simulink model "Flyback_Converter_Model_2014a"  (R2024a)
settings: Solver=ode3  StartTime=0.0  StopTime=0.25  FixedStep=1e-6  MaxStep=1e-4  RelTol=1e-4
libraries: spsSeriesRLCBranchLib x2, spsCurrentMeasurementLib x2, spsVoltageMeasurementLib x2, spsDiodeLib x1, spsMultimeterLib x1, spsMosfetLib x1, spsLinearTransformerLib x1, spsDCVoltageSourceLib x1, sps_lib x1
settings Model: Creator=A0109971  LastModifiedBy=DELL
settings SolverCC: AlgebraicLoopSolver=TrustRegion
settings DataIOCC: SaveFormat=StructureWithTime  ReturnWorkspaceOutputs=off
settings OptimizationCC: LifeSpan=inf
settings DebuggingCC: UnconnectedInputMsg=warning  UnconnectedOutputMsg=warning  UnconnectedLineMsg=warning  SFExecutionAtInitializationDiag=none  ArithmeticOperatorsInVariantConditions=warning
settings HardwareCC: ProdBitPerSizeT=32  ProdBitPerPtrDiffT=32  ProdWordSize=32  ProdHWDeviceType=Specified
settings SFSimCC: SimUseLocalCustomCode=off  CustomCodeUndefinedFunction=UseInterfaceOnly
settings RTWCC: RTWUseLocalCustomCode=off  GPUComputeCapability=3.5
settings CodeAppCC: StateflowObjectComments=on
settings SimscapeCC: SimscapeNormalizeSystem=off

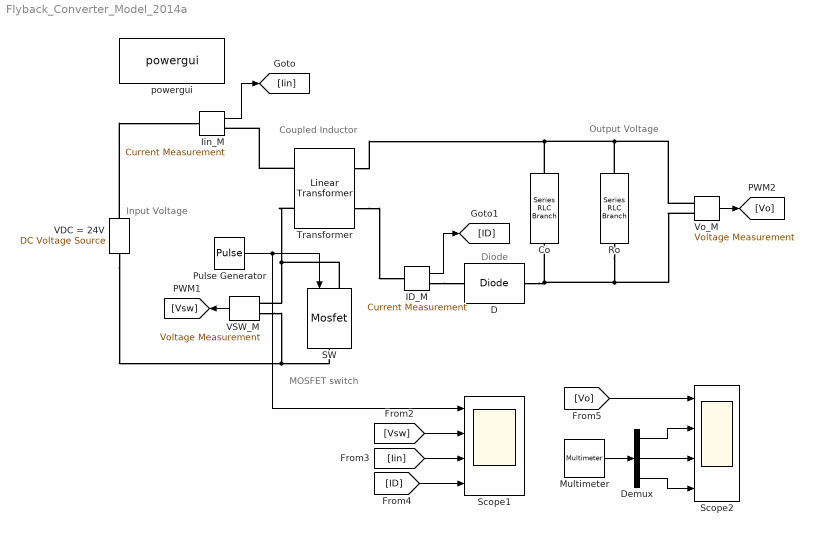
== system Flyback_Converter_Model_2014a ==
  note: Coupled Inductor
  note: Input Voltage
  note: MOSFET switch
  note: Diode
  note: Output Voltage
  Co : spsSeriesRLCBranchLib/Series RLC Branch  LConnTagsString=__new0  RConnTagsString=__new0  BranchType=C  Resistance=1  Inductance=1e-3  SetiL0=off  InitialCurrent=0  Capacitance=347e-6  Setx0=off  InitialVoltage=0  Measurements=None
  D : spsDiodeLib/Diode  Ron=1e-5  Lon=0  Vf=0  IC=0  UseSnubber=off  Rs=500*inf  Cs=250e-9  Measurements=off
  Demux : Demux  Outputs=3
  ID_M : spsCurrentMeasurementLib/Current Measurement  PhasorSimulation=off  OutputType=Complex  PSBequivalent=0
  Iin_M : spsCurrentMeasurementLib/Current Measurement  PhasorSimulation=off  OutputType=Complex  PSBequivalent=0
  Multimeter : spsMultimeterLib/Multimeter  L=8  sel=[3 7 1]  Gain=[1 1 1]  OutputType=Complex  PlotAtSimulationStop=off  PhasorSimulation=off
  Pulse Generator : DiscretePulseGenerator  PulseType=Time based  Period=20e-6  PulseWidth=50
  Ro : spsSeriesRLCBranchLib/Series RLC Branch  LConnTagsString=__new0  RConnTagsString=__new0  BranchType=R  Resistance=2.88  Inductance=1e-3  SetiL0=off  InitialCurrent=0  Capacitance=1e-6  Setx0=off  InitialVoltage=0  Measurements=Branch current
  SW : spsMosfetLib/Mosfet  Ron=1e-5  Lon=0  Rd=0.01  Vfd=0  IC=0  Rs=1e5  Cs=inf  Measurements=off
  Scope1 : Scope  NumInputPorts=4
  Scope2 : Scope  NumInputPorts=4
  Transformer : spsLinearTransformerLib/Linear Transformer  UNITS=SI  NominalPower=[ 50 50e3 ]  winding1=[24 0 0]  winding2=[12 0 0]  ThreeWindings=off  winding3=[3.15e+05 315.06 8.8673e-08]  RmLm=[1e6 192e-6]  Measurements=All voltages and currents  DataType=on
  VDC = 24V : spsDCVoltageSourceLib/DC Voltage Source  Amplitude=24  Measurements=None
  VSW_M : spsVoltageMeasurementLib/Voltage Measurement  PhasorSimulation=off  OutputType=Complex  PSBequivalent=0
  Vo_M : spsVoltageMeasurementLib/Voltage Measurement  PhasorSimulation=off  OutputType=Complex  PSBequivalent=0
  powergui : sps_lib/powergui  Priority=1  SimulationMode=Discrete  SampleTime=1e-6  frequency=60  Iterations=50  frequencyindice=0  Pbase=100e6  ErrMax=1e-4  UnitsV=kV  UnitsW=MW  buscounter=0  FunctionMessages=off  echomessages=off  EnableUseOfTLC=off  CurrentSourceSwitches=off  DisableSnubberDevices=off  DisableRonSwitches=off  DisableVfSwitches=off  DisplayEquations=off  AutomaticDiscreteSolvers=off  SolverType=Tustin/Backward Euler (TBE)  Interpol=off  ExternalGateDelay=off  methode=off  Ts=100  x0status=blocks  SPID=off  SwTol=0  HookPort=off  NonlinearTolerance=1e-4  nMaxIteration=100  ContinueOnMaxIteration=off  RestoreLinks=warning  ResistiveCurrentMeasurement=off  Frange=[0:2:500]  Ylog=off  Xlog=on  ShowGrid=off  save=off  variable=ZData  structure=0  ZoomFFT=off  StartTime=0.0  cycles=1  DisplayStyle=1  fundamental=60  FreqAxis=off  MaxFrequency=1000  frequencyindicesteady=1  RmsSteady=1  display=off
  wires:
  Pulse Generator/1 -> Scope1/1, SW/1
  VSW_M/1 -> [Vsw]
  [Vsw] -> Scope1/2
  Iin_M/1 -> [Iin]
  [Iin] -> Scope1/3
  Vo_M/1 -> [Vo]
  [ID] -> Scope1/4
  ID_M/1 -> [ID]
  [Vo] -> Scope2/1
  Demux/2 -> Scope2/3
  Demux/1 -> Scope2/2
  Demux/3 -> Scope2/4
  Multimeter/1 -> Demux/1
  connections:
  SW/LConn1 -- Transformer/LConn2 -- VSW_M/LConn1
  VDC = 24V/LConn1 -- VSW_M/LConn2 -- SW/RConn1
  D/RConn1 -- Vo_M/LConn1 -- Ro/LConn1 -- Co/LConn1
  Ro/RConn1 -- Vo_M/LConn2 -- Co/RConn1 -- Transformer/RConn1
  VDC = 24V/RConn1 -- Iin_M/LConn1
  ID_M/RConn1 -- D/LConn1
  Transformer/RConn2 -- ID_M/LConn1
  Transformer/LConn1 -- Iin_M/RConn1
